simulink model "benchmark_16bus_base_scenario"  (R2021a)
settings: Solver=ode4  StartTime=0.0  StopTime=5  FixedStep=Ts  MaxStep=50e-6  RelTol=1e-3
values from neighbouring files (symbols this model uses):
  Ctrl_Delay = 100e-6    (= 0.0001)    [init_anon.m]
  Pnom1 = 1330e6    (= 1330000000)    [init_anon.m]
  Pnom3 = 1e9    (= 1000000000)    [init_anon.m]
  Pnom4 = 64.4e6    (= 64400000)    [init_anon.m]
  Pnom5 = 19e6    (= 19000000)    [init_anon.m]
  Pnom6 = 450e6    (= 450000000)    [init_anon.m]
  Snom1 = 1e6*sqrt(1330^2 + (0.3*1330)^2)    [init_anon.m]
  Snom3 = 1044e6    (= 1044000000)    [init_anon.m]
  Snom4 = 1e6*sqrt(64.4^2 + (0.3*64.4)^2)    [init_anon.m]
  Snom5 = 1e6*sqrt(19^2 + (0.3*19)^2)    [init_anon.m]
  Snom6 = 1e6*sqrt(450^2 + (0.3*450)^2)    [init_anon.m]
  Ts = 5e-6    (= 5e-06)    [init_anon.m]
  wb = 2*pi*50    (= 314.159265359)    [init_anon.m]
  wcc = 1200    [init_anon.m]
  wlpf = 300    [init_anon.m]
  wp = 10    [init_anon.m]
  wv = 50    [init_anon.m]
  Zb = Ub^2/Sb    [init_anon.m]
undefined symbols (not defined in the file or in its folder): fb, Ib2, Ki_CC, Ki_i, Kp_CC, Kp_i, Kp_Rvi_pu, Lc_eq, Lf_pu, Rc_eq, Sb, Va0, Vb0, Vb1, Vb2, Vc0, Vm0, Vm0_d, Vm0_q, VSC01_id0, Vvsc0
libraries: spsGroundLib x135, spsParallelRLCBranchLib x132, Control_Lib x120, spsSeriesRLCBranchLib x66, spsThreePhaseSourceLib x22, spsThreePhaseBreakerLib x20, eeGeneralControl x20, slpidlib x15, spsLoadFlowBusLib x13, spsThreePhaseVIMeasurementLib x12, spsThreePhaseTransformerTwoWindingsLib x11, spsUniversalBridgeLib x10
(part 3 of 9)

== system benchmark_16bus_base_scenario/Subsystem15 ==
  Ground{,1..5} (6 alike) : spsGroundLib/Ground  LConnTagsString=a
  Parallel RLC Branch{,1..5} (6 alike) : spsParallelRLCBranchLib/Parallel RLC Branch  LConnTagsString=a  RConnTagsString=__new0  BranchType=C  Resistance=1  Inductance=1e-3  SetiL0=off  InitialCurrent=0  Capacitance=C  Setx0=off  InitialVoltage=0  Measurements=None
  Series RLC Branch : spsSeriesRLCBranchLib/Series RLC Branch  LConnTagsString=__new0  RConnTagsString=__new0  BranchType=RL  Resistance=R  Inductance=L  SetiL0=off  InitialCurrent=0  Capacitance=1e-6  Setx0=off  InitialVoltage=0  Measurements=None
  Series RLC Branch3 : spsSeriesRLCBranchLib/Series RLC Branch  LConnTagsString=__new0  RConnTagsString=__new0  BranchType=RL  Resistance=R  Inductance=L  SetiL0=off  InitialCurrent=0  Capacitance=1e-6  Setx0=off  InitialVoltage=0  Measurements=None
  Series RLC Branch6 : spsSeriesRLCBranchLib/Series RLC Branch  LConnTagsString=__new0  RConnTagsString=__new0  BranchType=RL  Resistance=R  Inductance=L  SetiL0=off  InitialCurrent=0  Capacitance=1e-6  Setx0=off  InitialVoltage=0  Measurements=None
  A : PMIOPort  Side=Left
  a : PMIOPort  Port=2  Side=Right
  B : PMIOPort  Port=3  Side=Left
  b : PMIOPort  Port=4  Side=Right
  C : PMIOPort  Port=5  Side=Left
  c : PMIOPort  Port=6  Side=Right
  connections:
  Ground5/LConn1 -- Parallel RLC Branch5/RConn1
  Ground4/LConn1 -- Parallel RLC Branch4/RConn1
  Series RLC Branch6/RConn1 -- Parallel RLC Branch5/LConn1 -- c/RConn1
  Series RLC Branch6/LConn1 -- Parallel RLC Branch4/LConn1 -- C/RConn1
  Ground3/LConn1 -- Parallel RLC Branch3/RConn1
  Ground2/LConn1 -- Parallel RLC Branch2/RConn1
  Series RLC Branch3/RConn1 -- Parallel RLC Branch3/LConn1 -- b/RConn1
  Series RLC Branch3/LConn1 -- Parallel RLC Branch2/LConn1 -- B/RConn1
  Parallel RLC Branch1/LConn1 -- a/RConn1 -- Series RLC Branch/RConn1
  Ground/LConn1 -- Parallel RLC Branch/RConn1
  Parallel RLC Branch/LConn1 -- A/RConn1 -- Series RLC Branch/LConn1
  Ground1/LConn1 -- Parallel RLC Branch1/RConn1

== system benchmark_16bus_base_scenario/Subsystem16 ==
  Ground{,1..5} (6 alike) : spsGroundLib/Ground  LConnTagsString=a
  Parallel RLC Branch{,1..5} (6 alike) : spsParallelRLCBranchLib/Parallel RLC Branch  LConnTagsString=a  RConnTagsString=__new0  BranchType=C  Resistance=1  Inductance=1e-3  SetiL0=off  InitialCurrent=0  Capacitance=C  Setx0=off  InitialVoltage=0  Measurements=None
  Series RLC Branch : spsSeriesRLCBranchLib/Series RLC Branch  LConnTagsString=__new0  RConnTagsString=__new0  BranchType=RL  Resistance=R  Inductance=L  SetiL0=off  InitialCurrent=0  Capacitance=1e-6  Setx0=off  InitialVoltage=0  Measurements=None
  Series RLC Branch3 : spsSeriesRLCBranchLib/Series RLC Branch  LConnTagsString=__new0  RConnTagsString=__new0  BranchType=RL  Resistance=R  Inductance=L  SetiL0=off  InitialCurrent=0  Capacitance=1e-6  Setx0=off  InitialVoltage=0  Measurements=None
  Series RLC Branch6 : spsSeriesRLCBranchLib/Series RLC Branch  LConnTagsString=__new0  RConnTagsString=__new0  BranchType=RL  Resistance=R  Inductance=L  SetiL0=off  InitialCurrent=0  Capacitance=1e-6  Setx0=off  InitialVoltage=0  Measurements=None
  A : PMIOPort  Side=Left
  a : PMIOPort  Port=2  Side=Right
  B : PMIOPort  Port=3  Side=Left
  b : PMIOPort  Port=4  Side=Right
  C : PMIOPort  Port=5  Side=Left
  c : PMIOPort  Port=6  Side=Right
  connections:
  Ground1/LConn1 -- Parallel RLC Branch1/RConn1
  Series RLC Branch/LConn1 -- A/RConn1 -- Parallel RLC Branch/LConn1
  Ground/LConn1 -- Parallel RLC Branch/RConn1
  Series RLC Branch/RConn1 -- a/RConn1 -- Parallel RLC Branch1/LConn1
  B/RConn1 -- Parallel RLC Branch2/LConn1 -- Series RLC Branch3/LConn1
  b/RConn1 -- Parallel RLC Branch3/LConn1 -- Series RLC Branch3/RConn1
  Ground2/LConn1 -- Parallel RLC Branch2/RConn1
  Ground3/LConn1 -- Parallel RLC Branch3/RConn1
  C/RConn1 -- Parallel RLC Branch4/LConn1 -- Series RLC Branch6/LConn1
  c/RConn1 -- Parallel RLC Branch5/LConn1 -- Series RLC Branch6/RConn1
  Ground4/LConn1 -- Parallel RLC Branch4/RConn1
  Ground5/LConn1 -- Parallel RLC Branch5/RConn1

== system benchmark_16bus_base_scenario/Subsystem17 ==
  Ground{,1..5} (6 alike) : spsGroundLib/Ground  LConnTagsString=a
  Parallel RLC Branch{,1..5} (6 alike) : spsParallelRLCBranchLib/Parallel RLC Branch  LConnTagsString=a  RConnTagsString=__new0  BranchType=C  Resistance=1  Inductance=1e-3  SetiL0=off  InitialCurrent=0  Capacitance=C  Setx0=off  InitialVoltage=0  Measurements=None
  Series RLC Branch : spsSeriesRLCBranchLib/Series RLC Branch  LConnTagsString=__new0  RConnTagsString=__new0  BranchType=RL  Resistance=R  Inductance=L  SetiL0=off  InitialCurrent=0  Capacitance=1e-6  Setx0=off  InitialVoltage=0  Measurements=None
  Series RLC Branch3 : spsSeriesRLCBranchLib/Series RLC Branch  LConnTagsString=__new0  RConnTagsString=__new0  BranchType=RL  Resistance=R  Inductance=L  SetiL0=off  InitialCurrent=0  Capacitance=1e-6  Setx0=off  InitialVoltage=0  Measurements=None
  Series RLC Branch6 : spsSeriesRLCBranchLib/Series RLC Branch  LConnTagsString=__new0  RConnTagsString=__new0  BranchType=RL  Resistance=R  Inductance=L  SetiL0=off  InitialCurrent=0  Capacitance=1e-6  Setx0=off  InitialVoltage=0  Measurements=None
  A : PMIOPort  Side=Left
  a : PMIOPort  Port=2  Side=Right
  B : PMIOPort  Port=3  Side=Left
  b : PMIOPort  Port=4  Side=Right
  C : PMIOPort  Port=5  Side=Left
  c : PMIOPort  Port=6  Side=Right
  connections:
  Ground5/LConn1 -- Parallel RLC Branch5/RConn1
  Ground4/LConn1 -- Parallel RLC Branch4/RConn1
  Series RLC Branch6/RConn1 -- Parallel RLC Branch5/LConn1 -- c/RConn1
  Series RLC Branch6/LConn1 -- Parallel RLC Branch4/LConn1 -- C/RConn1
  Ground3/LConn1 -- Parallel RLC Branch3/RConn1
  Ground2/LConn1 -- Parallel RLC Branch2/RConn1
  Series RLC Branch3/RConn1 -- Parallel RLC Branch3/LConn1 -- b/RConn1
  Series RLC Branch3/LConn1 -- Parallel RLC Branch2/LConn1 -- B/RConn1
  Parallel RLC Branch1/LConn1 -- a/RConn1 -- Series RLC Branch/RConn1
  Ground/LConn1 -- Parallel RLC Branch/RConn1
  Parallel RLC Branch/LConn1 -- A/RConn1 -- Series RLC Branch/LConn1
  Ground1/LConn1 -- Parallel RLC Branch1/RConn1

== system benchmark_16bus_base_scenario/Subsystem18 ==
  Ground{,1..5} (6 alike) : spsGroundLib/Ground  LConnTagsString=a
  Parallel RLC Branch{,1..5} (6 alike) : spsParallelRLCBranchLib/Parallel RLC Branch  LConnTagsString=a  RConnTagsString=__new0  BranchType=C  Resistance=1  Inductance=1e-3  SetiL0=off  InitialCurrent=0  Capacitance=C  Setx0=off  InitialVoltage=0  Measurements=None
  Series RLC Branch : spsSeriesRLCBranchLib/Series RLC Branch  LConnTagsString=__new0  RConnTagsString=__new0  BranchType=RL  Resistance=R  Inductance=L  SetiL0=off  InitialCurrent=0  Capacitance=1e-6  Setx0=off  InitialVoltage=0  Measurements=None
  Series RLC Branch3 : spsSeriesRLCBranchLib/Series RLC Branch  LConnTagsString=__new0  RConnTagsString=__new0  BranchType=RL  Resistance=R  Inductance=L  SetiL0=off  InitialCurrent=0  Capacitance=1e-6  Setx0=off  InitialVoltage=0  Measurements=None
  Series RLC Branch6 : spsSeriesRLCBranchLib/Series RLC Branch  LConnTagsString=__new0  RConnTagsString=__new0  BranchType=RL  Resistance=R  Inductance=L  SetiL0=off  InitialCurrent=0  Capacitance=1e-6  Setx0=off  InitialVoltage=0  Measurements=None
  A : PMIOPort  Side=Left
  a : PMIOPort  Port=2  Side=Right
  B : PMIOPort  Port=3  Side=Left
  b : PMIOPort  Port=4  Side=Right
  C : PMIOPort  Port=5  Side=Left
  c : PMIOPort  Port=6  Side=Right
  connections:
  Ground5/LConn1 -- Parallel RLC Branch5/RConn1
  Ground4/LConn1 -- Parallel RLC Branch4/RConn1
  Series RLC Branch6/RConn1 -- Parallel RLC Branch5/LConn1 -- c/RConn1
  Series RLC Branch6/LConn1 -- Parallel RLC Branch4/LConn1 -- C/RConn1
  Ground3/LConn1 -- Parallel RLC Branch3/RConn1
  Ground2/LConn1 -- Parallel RLC Branch2/RConn1
  Series RLC Branch3/RConn1 -- Parallel RLC Branch3/LConn1 -- b/RConn1
  Series RLC Branch3/LConn1 -- Parallel RLC Branch2/LConn1 -- B/RConn1
  Parallel RLC Branch1/LConn1 -- a/RConn1 -- Series RLC Branch/RConn1
  Ground/LConn1 -- Parallel RLC Branch/RConn1
  Parallel RLC Branch/LConn1 -- A/RConn1 -- Series RLC Branch/LConn1
  Ground1/LConn1 -- Parallel RLC Branch1/RConn1

== system benchmark_16bus_base_scenario/Subsystem19 ==
  Ground{,1..5} (6 alike) : spsGroundLib/Ground  LConnTagsString=a
  Parallel RLC Branch{,1..5} (6 alike) : spsParallelRLCBranchLib/Parallel RLC Branch  LConnTagsString=a  RConnTagsString=__new0  BranchType=C  Resistance=1  Inductance=1e-3  SetiL0=off  InitialCurrent=0  Capacitance=C  Setx0=off  InitialVoltage=0  Measurements=None
  Series RLC Branch : spsSeriesRLCBranchLib/Series RLC Branch  LConnTagsString=__new0  RConnTagsString=__new0  BranchType=RL  Resistance=R  Inductance=L  SetiL0=off  InitialCurrent=0  Capacitance=1e-6  Setx0=off  InitialVoltage=0  Measurements=None
  Series RLC Branch3 : spsSeriesRLCBranchLib/Series RLC Branch  LConnTagsString=__new0  RConnTagsString=__new0  BranchType=RL  Resistance=R  Inductance=L  SetiL0=off  InitialCurrent=0  Capacitance=1e-6  Setx0=off  InitialVoltage=0  Measurements=None
  Series RLC Branch6 : spsSeriesRLCBranchLib/Series RLC Branch  LConnTagsString=__new0  RConnTagsString=__new0  BranchType=RL  Resistance=R  Inductance=L  SetiL0=off  InitialCurrent=0  Capacitance=1e-6  Setx0=off  InitialVoltage=0  Measurements=None
  A : PMIOPort  Side=Left
  a : PMIOPort  Port=2  Side=Right
  B : PMIOPort  Port=3  Side=Left
  b : PMIOPort  Port=4  Side=Right
  C : PMIOPort  Port=5  Side=Left
  c : PMIOPort  Port=6  Side=Right
  connections:
  Ground1/LConn1 -- Parallel RLC Branch1/RConn1
  Series RLC Branch/LConn1 -- A/RConn1 -- Parallel RLC Branch/LConn1
  Ground/LConn1 -- Parallel RLC Branch/RConn1
  Series RLC Branch/RConn1 -- a/RConn1 -- Parallel RLC Branch1/LConn1
  B/RConn1 -- Parallel RLC Branch2/LConn1 -- Series RLC Branch3/LConn1
  b/RConn1 -- Parallel RLC Branch3/LConn1 -- Series RLC Branch3/RConn1
  Ground2/LConn1 -- Parallel RLC Branch2/RConn1
  Ground3/LConn1 -- Parallel RLC Branch3/RConn1
  C/RConn1 -- Parallel RLC Branch4/LConn1 -- Series RLC Branch6/LConn1
  c/RConn1 -- Parallel RLC Branch5/LConn1 -- Series RLC Branch6/RConn1
  Ground4/LConn1 -- Parallel RLC Branch4/RConn1
  Ground5/LConn1 -- Parallel RLC Branch5/RConn1

== system benchmark_16bus_base_scenario/Subsystem20 ==
  Ground{,1..5} (6 alike) : spsGroundLib/Ground  LConnTagsString=a
  Parallel RLC Branch{,1..5} (6 alike) : spsParallelRLCBranchLib/Parallel RLC Branch  LConnTagsString=a  RConnTagsString=__new0  BranchType=C  Resistance=1  Inductance=1e-3  SetiL0=off  InitialCurrent=0  Capacitance=C  Setx0=off  InitialVoltage=0  Measurements=None
  Series RLC Branch : spsSeriesRLCBranchLib/Series RLC Branch  LConnTagsString=__new0  RConnTagsString=__new0  BranchType=RL  Resistance=R  Inductance=L  SetiL0=off  InitialCurrent=0  Capacitance=1e-6  Setx0=off  InitialVoltage=0  Measurements=None
  Series RLC Branch3 : spsSeriesRLCBranchLib/Series RLC Branch  LConnTagsString=__new0  RConnTagsString=__new0  BranchType=RL  Resistance=R  Inductance=L  SetiL0=off  InitialCurrent=0  Capacitance=1e-6  Setx0=off  InitialVoltage=0  Measurements=None
  Series RLC Branch6 : spsSeriesRLCBranchLib/Series RLC Branch  LConnTagsString=__new0  RConnTagsString=__new0  BranchType=RL  Resistance=R  Inductance=L  SetiL0=off  InitialCurrent=0  Capacitance=1e-6  Setx0=off  InitialVoltage=0  Measurements=None
  A : PMIOPort  Side=Left
  a : PMIOPort  Port=2  Side=Right
  B : PMIOPort  Port=3  Side=Left
  b : PMIOPort  Port=4  Side=Right
  C : PMIOPort  Port=5  Side=Left
  c : PMIOPort  Port=6  Side=Right
  connections:
  Ground1/LConn1 -- Parallel RLC Branch1/RConn1
  Series RLC Branch/LConn1 -- A/RConn1 -- Parallel RLC Branch/LConn1
  Ground/LConn1 -- Parallel RLC Branch/RConn1
  Series RLC Branch/RConn1 -- a/RConn1 -- Parallel RLC Branch1/LConn1
  B/RConn1 -- Parallel RLC Branch2/LConn1 -- Series RLC Branch3/LConn1
  b/RConn1 -- Parallel RLC Branch3/LConn1 -- Series RLC Branch3/RConn1
  Ground2/LConn1 -- Parallel RLC Branch2/RConn1
  Ground3/LConn1 -- Parallel RLC Branch3/RConn1
  C/RConn1 -- Parallel RLC Branch4/LConn1 -- Series RLC Branch6/LConn1
  c/RConn1 -- Parallel RLC Branch5/LConn1 -- Series RLC Branch6/RConn1
  Ground4/LConn1 -- Parallel RLC Branch4/RConn1
  Ground5/LConn1 -- Parallel RLC Branch5/RConn1

== system benchmark_16bus_base_scenario/Subsystem21 ==
  Ground{,1..5} (6 alike) : spsGroundLib/Ground  LConnTagsString=a
  Parallel RLC Branch{,1..5} (6 alike) : spsParallelRLCBranchLib/Parallel RLC Branch  LConnTagsString=a  RConnTagsString=__new0  BranchType=C  Resistance=1  Inductance=1e-3  SetiL0=off  InitialCurrent=0  Capacitance=C  Setx0=off  InitialVoltage=0  Measurements=None
  Series RLC Branch : spsSeriesRLCBranchLib/Series RLC Branch  LConnTagsString=__new0  RConnTagsString=__new0  BranchType=RL  Resistance=R  Inductance=L  SetiL0=off  InitialCurrent=0  Capacitance=1e-6  Setx0=off  InitialVoltage=0  Measurements=None
  Series RLC Branch3 : spsSeriesRLCBranchLib/Series RLC Branch  LConnTagsString=__new0  RConnTagsString=__new0  BranchType=RL  Resistance=R  Inductance=L  SetiL0=off  InitialCurrent=0  Capacitance=1e-6  Setx0=off  InitialVoltage=0  Measurements=None
  Series RLC Branch6 : spsSeriesRLCBranchLib/Series RLC Branch  LConnTagsString=__new0  RConnTagsString=__new0  BranchType=RL  Resistance=R  Inductance=L  SetiL0=off  InitialCurrent=0  Capacitance=1e-6  Setx0=off  InitialVoltage=0  Measurements=None
  A : PMIOPort  Side=Left
  a : PMIOPort  Port=2  Side=Right
  B : PMIOPort  Port=3  Side=Left
  b : PMIOPort  Port=4  Side=Right
  C : PMIOPort  Port=5  Side=Left
  c : PMIOPort  Port=6  Side=Right
  connections:
  Ground5/LConn1 -- Parallel RLC Branch5/RConn1
  Ground4/LConn1 -- Parallel RLC Branch4/RConn1
  Series RLC Branch6/RConn1 -- Parallel RLC Branch5/LConn1 -- c/RConn1
  Series RLC Branch6/LConn1 -- Parallel RLC Branch4/LConn1 -- C/RConn1
  Ground3/LConn1 -- Parallel RLC Branch3/RConn1
  Ground2/LConn1 -- Parallel RLC Branch2/RConn1
  Series RLC Branch3/RConn1 -- Parallel RLC Branch3/LConn1 -- b/RConn1
  Series RLC Branch3/LConn1 -- Parallel RLC Branch2/LConn1 -- B/RConn1
  Parallel RLC Branch1/LConn1 -- a/RConn1 -- Series RLC Branch/RConn1
  Ground/LConn1 -- Parallel RLC Branch/RConn1
  Parallel RLC Branch/LConn1 -- A/RConn1 -- Series RLC Branch/LConn1
  Ground1/LConn1 -- Parallel RLC Branch1/RConn1

== system benchmark_16bus_base_scenario/Subsystem22 ==
  Ground{,1..5} (6 alike) : spsGroundLib/Ground  LConnTagsString=a
  Parallel RLC Branch{,1..5} (6 alike) : spsParallelRLCBranchLib/Parallel RLC Branch  LConnTagsString=a  RConnTagsString=__new0  BranchType=C  Resistance=1  Inductance=1e-3  SetiL0=off  InitialCurrent=0  Capacitance=C  Setx0=off  InitialVoltage=0  Measurements=None
  Series RLC Branch : spsSeriesRLCBranchLib/Series RLC Branch  LConnTagsString=__new0  RConnTagsString=__new0  BranchType=RL  Resistance=R  Inductance=L  SetiL0=off  InitialCurrent=0  Capacitance=1e-6  Setx0=off  InitialVoltage=0  Measurements=None
  Series RLC Branch3 : spsSeriesRLCBranchLib/Series RLC Branch  LConnTagsString=__new0  RConnTagsString=__new0  BranchType=RL  Resistance=R  Inductance=L  SetiL0=off  InitialCurrent=0  Capacitance=1e-6  Setx0=off  InitialVoltage=0  Measurements=None
  Series RLC Branch6 : spsSeriesRLCBranchLib/Series RLC Branch  LConnTagsString=__new0  RConnTagsString=__new0  BranchType=RL  Resistance=R  Inductance=L  SetiL0=off  InitialCurrent=0  Capacitance=1e-6  Setx0=off  InitialVoltage=0  Measurements=None
  A : PMIOPort  Side=Left
  a : PMIOPort  Port=2  Side=Right
  B : PMIOPort  Port=3  Side=Left
  b : PMIOPort  Port=4  Side=Right
  C : PMIOPort  Port=5  Side=Left
  c : PMIOPort  Port=6  Side=Right
  connections:
  Ground5/LConn1 -- Parallel RLC Branch5/RConn1
  Ground4/LConn1 -- Parallel RLC Branch4/RConn1
  Series RLC Branch6/RConn1 -- Parallel RLC Branch5/LConn1 -- c/RConn1
  Series RLC Branch6/LConn1 -- Parallel RLC Branch4/LConn1 -- C/RConn1
  Ground3/LConn1 -- Parallel RLC Branch3/RConn1
  Ground2/LConn1 -- Parallel RLC Branch2/RConn1
  Series RLC Branch3/RConn1 -- Parallel RLC Branch3/LConn1 -- b/RConn1
  Series RLC Branch3/LConn1 -- Parallel RLC Branch2/LConn1 -- B/RConn1
  Parallel RLC Branch1/LConn1 -- a/RConn1 -- Series RLC Branch/RConn1
  Ground/LConn1 -- Parallel RLC Branch/RConn1
  Parallel RLC Branch/LConn1 -- A/RConn1 -- Series RLC Branch/LConn1
  Ground1/LConn1 -- Parallel RLC Branch1/RConn1

== system benchmark_16bus_base_scenario/Subsystem23 ==
  Ground{,1..5} (6 alike) : spsGroundLib/Ground  LConnTagsString=a
  Parallel RLC Branch{,1..5} (6 alike) : spsParallelRLCBranchLib/Parallel RLC Branch  LConnTagsString=a  RConnTagsString=__new0  BranchType=C  Resistance=1  Inductance=1e-3  SetiL0=off  InitialCurrent=0  Capacitance=C  Setx0=off  InitialVoltage=0  Measurements=None
  Series RLC Branch : spsSeriesRLCBranchLib/Series RLC Branch  LConnTagsString=__new0  RConnTagsString=__new0  BranchType=RL  Resistance=R  Inductance=L  SetiL0=off  InitialCurrent=0  Capacitance=1e-6  Setx0=off  InitialVoltage=0  Measurements=None
  Series RLC Branch3 : spsSeriesRLCBranchLib/Series RLC Branch  LConnTagsString=__new0  RConnTagsString=__new0  BranchType=RL  Resistance=R  Inductance=L  SetiL0=off  InitialCurrent=0  Capacitance=1e-6  Setx0=off  InitialVoltage=0  Measurements=None
  Series RLC Branch6 : spsSeriesRLCBranchLib/Series RLC Branch  LConnTagsString=__new0  RConnTagsString=__new0  BranchType=RL  Resistance=R  Inductance=L  SetiL0=off  InitialCurrent=0  Capacitance=1e-6  Setx0=off  InitialVoltage=0  Measurements=None
  A : PMIOPort  Side=Left
  a : PMIOPort  Port=2  Side=Right
  B : PMIOPort  Port=3  Side=Left
  b : PMIOPort  Port=4  Side=Right
  C : PMIOPort  Port=5  Side=Left
  c : PMIOPort  Port=6  Side=Right
  connections:
  Ground1/LConn1 -- Parallel RLC Branch1/RConn1
  Series RLC Branch/LConn1 -- A/RConn1 -- Parallel RLC Branch/LConn1
  Ground/LConn1 -- Parallel RLC Branch/RConn1
  Series RLC Branch/RConn1 -- a/RConn1 -- Parallel RLC Branch1/LConn1
  B/RConn1 -- Parallel RLC Branch2/LConn1 -- Series RLC Branch3/LConn1
  b/RConn1 -- Parallel RLC Branch3/LConn1 -- Series RLC Branch3/RConn1
  Ground2/LConn1 -- Parallel RLC Branch2/RConn1
  Ground3/LConn1 -- Parallel RLC Branch3/RConn1
  C/RConn1 -- Parallel RLC Branch4/LConn1 -- Series RLC Branch6/LConn1
  c/RConn1 -- Parallel RLC Branch5/LConn1 -- Series RLC Branch6/RConn1
  Ground4/LConn1 -- Parallel RLC Branch4/RConn1
  Ground5/LConn1 -- Parallel RLC Branch5/RConn1

== system benchmark_16bus_base_scenario/Subsystem24 ==
  Ground{,1..5} (6 alike) : spsGroundLib/Ground  LConnTagsString=a
  Parallel RLC Branch{,1..5} (6 alike) : spsParallelRLCBranchLib/Parallel RLC Branch  LConnTagsString=a  RConnTagsString=__new0  BranchType=C  Resistance=1  Inductance=1e-3  SetiL0=off  InitialCurrent=0  Capacitance=C  Setx0=off  InitialVoltage=0  Measurements=None
  Series RLC Branch : spsSeriesRLCBranchLib/Series RLC Branch  LConnTagsString=__new0  RConnTagsString=__new0  BranchType=RL  Resistance=R  Inductance=L  SetiL0=off  InitialCurrent=0  Capacitance=1e-6  Setx0=off  InitialVoltage=0  Measurements=None
  Series RLC Branch3 : spsSeriesRLCBranchLib/Series RLC Branch  LConnTagsString=__new0  RConnTagsString=__new0  BranchType=RL  Resistance=R  Inductance=L  SetiL0=off  InitialCurrent=0  Capacitance=1e-6  Setx0=off  InitialVoltage=0  Measurements=None
  Series RLC Branch6 : spsSeriesRLCBranchLib/Series RLC Branch  LConnTagsString=__new0  RConnTagsString=__new0  BranchType=RL  Resistance=R  Inductance=L  SetiL0=off  InitialCurrent=0  Capacitance=1e-6  Setx0=off  InitialVoltage=0  Measurements=None
  A : PMIOPort  Side=Left
  a : PMIOPort  Port=2  Side=Right
  B : PMIOPort  Port=3  Side=Left
  b : PMIOPort  Port=4  Side=Right
  C : PMIOPort  Port=5  Side=Left
  c : PMIOPort  Port=6  Side=Right
  connections:
  Ground5/LConn1 -- Parallel RLC Branch5/RConn1
  Ground4/LConn1 -- Parallel RLC Branch4/RConn1
  Series RLC Branch6/RConn1 -- Parallel RLC Branch5/LConn1 -- c/RConn1
  Series RLC Branch6/LConn1 -- Parallel RLC Branch4/LConn1 -- C/RConn1
  Ground3/LConn1 -- Parallel RLC Branch3/RConn1
  Ground2/LConn1 -- Parallel RLC Branch2/RConn1
  Series RLC Branch3/RConn1 -- Parallel RLC Branch3/LConn1 -- b/RConn1
  Series RLC Branch3/LConn1 -- Parallel RLC Branch2/LConn1 -- B/RConn1
  Parallel RLC Branch1/LConn1 -- a/RConn1 -- Series RLC Branch/RConn1
  Ground/LConn1 -- Parallel RLC Branch/RConn1
  Parallel RLC Branch/LConn1 -- A/RConn1 -- Series RLC Branch/LConn1
  Ground1/LConn1 -- Parallel RLC Branch1/RConn1

== system benchmark_16bus_base_scenario/Subsystem25 ==
  Ground{,1..5} (6 alike) : spsGroundLib/Ground  LConnTagsString=a
  Parallel RLC Branch{,1..5} (6 alike) : spsParallelRLCBranchLib/Parallel RLC Branch  LConnTagsString=a  RConnTagsString=__new0  BranchType=C  Resistance=1  Inductance=1e-3  SetiL0=off  InitialCurrent=0  Capacitance=C  Setx0=off  InitialVoltage=0  Measurements=None
  Series RLC Branch : spsSeriesRLCBranchLib/Series RLC Branch  LConnTagsString=__new0  RConnTagsString=__new0  BranchType=RL  Resistance=R  Inductance=L  SetiL0=off  InitialCurrent=0  Capacitance=1e-6  Setx0=off  InitialVoltage=0  Measurements=None
  Series RLC Branch3 : spsSeriesRLCBranchLib/Series RLC Branch  LConnTagsString=__new0  RConnTagsString=__new0  BranchType=RL  Resistance=R  Inductance=L  SetiL0=off  InitialCurrent=0  Capacitance=1e-6  Setx0=off  InitialVoltage=0  Measurements=None
  Series RLC Branch6 : spsSeriesRLCBranchLib/Series RLC Branch  LConnTagsString=__new0  RConnTagsString=__new0  BranchType=RL  Resistance=R  Inductance=L  SetiL0=off  InitialCurrent=0  Capacitance=1e-6  Setx0=off  InitialVoltage=0  Measurements=None
  A : PMIOPort  Side=Left
  a : PMIOPort  Port=2  Side=Right
  B : PMIOPort  Port=3  Side=Left
  b : PMIOPort  Port=4  Side=Right
  C : PMIOPort  Port=5  Side=Left
  c : PMIOPort  Port=6  Side=Right
  connections:
  Ground1/LConn1 -- Parallel RLC Branch1/RConn1
  Series RLC Branch/LConn1 -- A/RConn1 -- Parallel RLC Branch/LConn1
  Ground/LConn1 -- Parallel RLC Branch/RConn1
  Series RLC Branch/RConn1 -- a/RConn1 -- Parallel RLC Branch1/LConn1
  B/RConn1 -- Parallel RLC Branch2/LConn1 -- Series RLC Branch3/LConn1
  b/RConn1 -- Parallel RLC Branch3/LConn1 -- Series RLC Branch3/RConn1
  Ground2/LConn1 -- Parallel RLC Branch2/RConn1
  Ground3/LConn1 -- Parallel RLC Branch3/RConn1
  C/RConn1 -- Parallel RLC Branch4/LConn1 -- Series RLC Branch6/LConn1
  c/RConn1 -- Parallel RLC Branch5/LConn1 -- Series RLC Branch6/RConn1
  Ground4/LConn1 -- Parallel RLC Branch4/RConn1
  Ground5/LConn1 -- Parallel RLC Branch5/RConn1

== system benchmark_16bus_base_scenario/Subsystem26 ==
  Ground{,1..5} (6 alike) : spsGroundLib/Ground  LConnTagsString=a
  Parallel RLC Branch{,1..5} (6 alike) : spsParallelRLCBranchLib/Parallel RLC Branch  LConnTagsString=a  RConnTagsString=__new0  BranchType=C  Resistance=1  Inductance=1e-3  SetiL0=off  InitialCurrent=0  Capacitance=C  Setx0=off  InitialVoltage=0  Measurements=None
  Series RLC Branch : spsSeriesRLCBranchLib/Series RLC Branch  LConnTagsString=__new0  RConnTagsString=__new0  BranchType=RL  Resistance=R  Inductance=L  SetiL0=off  InitialCurrent=0  Capacitance=1e-6  Setx0=off  InitialVoltage=0  Measurements=None
  Series RLC Branch3 : spsSeriesRLCBranchLib/Series RLC Branch  LConnTagsString=__new0  RConnTagsString=__new0  BranchType=RL  Resistance=R  Inductance=L  SetiL0=off  InitialCurrent=0  Capacitance=1e-6  Setx0=off  InitialVoltage=0  Measurements=None
  Series RLC Branch6 : spsSeriesRLCBranchLib/Series RLC Branch  LConnTagsString=__new0  RConnTagsString=__new0  BranchType=RL  Resistance=R  Inductance=L  SetiL0=off  InitialCurrent=0  Capacitance=1e-6  Setx0=off  InitialVoltage=0  Measurements=None
  A : PMIOPort  Side=Left
  a : PMIOPort  Port=2  Side=Right
  B : PMIOPort  Port=3  Side=Left
  b : PMIOPort  Port=4  Side=Right
  C : PMIOPort  Port=5  Side=Left
  c : PMIOPort  Port=6  Side=Right
  connections:
  Ground5/LConn1 -- Parallel RLC Branch5/RConn1
  Ground4/LConn1 -- Parallel RLC Branch4/RConn1
  Series RLC Branch6/RConn1 -- Parallel RLC Branch5/LConn1 -- c/RConn1
  Series RLC Branch6/LConn1 -- Parallel RLC Branch4/LConn1 -- C/RConn1
  Ground3/LConn1 -- Parallel RLC Branch3/RConn1
  Ground2/LConn1 -- Parallel RLC Branch2/RConn1
  Series RLC Branch3/RConn1 -- Parallel RLC Branch3/LConn1 -- b/RConn1
  Series RLC Branch3/LConn1 -- Parallel RLC Branch2/LConn1 -- B/RConn1
  Parallel RLC Branch1/LConn1 -- a/RConn1 -- Series RLC Branch/RConn1
  Ground/LConn1 -- Parallel RLC Branch/RConn1
  Parallel RLC Branch/LConn1 -- A/RConn1 -- Series RLC Branch/LConn1
  Ground1/LConn1 -- Parallel RLC Branch1/RConn1

== system benchmark_16bus_base_scenario/Subsystem27 ==
  Ground{,1..5} (6 alike) : spsGroundLib/Ground  LConnTagsString=a
  Parallel RLC Branch{,1..5} (6 alike) : spsParallelRLCBranchLib/Parallel RLC Branch  LConnTagsString=a  RConnTagsString=__new0  BranchType=C  Resistance=1  Inductance=1e-3  SetiL0=off  InitialCurrent=0  Capacitance=C  Setx0=off  InitialVoltage=0  Measurements=None
  Series RLC Branch : spsSeriesRLCBranchLib/Series RLC Branch  LConnTagsString=__new0  RConnTagsString=__new0  BranchType=RL  Resistance=R  Inductance=L  SetiL0=off  InitialCurrent=0  Capacitance=1e-6  Setx0=off  InitialVoltage=0  Measurements=None
  Series RLC Branch3 : spsSeriesRLCBranchLib/Series RLC Branch  LConnTagsString=__new0  RConnTagsString=__new0  BranchType=RL  Resistance=R  Inductance=L  SetiL0=off  InitialCurrent=0  Capacitance=1e-6  Setx0=off  InitialVoltage=0  Measurements=None
  Series RLC Branch6 : spsSeriesRLCBranchLib/Series RLC Branch  LConnTagsString=__new0  RConnTagsString=__new0  BranchType=RL  Resistance=R  Inductance=L  SetiL0=off  InitialCurrent=0  Capacitance=1e-6  Setx0=off  InitialVoltage=0  Measurements=None
  A : PMIOPort  Side=Left
  a : PMIOPort  Port=2  Side=Right
  B : PMIOPort  Port=3  Side=Left
  b : PMIOPort  Port=4  Side=Right
  C : PMIOPort  Port=5  Side=Left
  c : PMIOPort  Port=6  Side=Right
  connections:
  Ground1/LConn1 -- Parallel RLC Branch1/RConn1
  Series RLC Branch/LConn1 -- A/RConn1 -- Parallel RLC Branch/LConn1
  Ground/LConn1 -- Parallel RLC Branch/RConn1
  Series RLC Branch/RConn1 -- a/RConn1 -- Parallel RLC Branch1/LConn1
  B/RConn1 -- Parallel RLC Branch2/LConn1 -- Series RLC Branch3/LConn1
  b/RConn1 -- Parallel RLC Branch3/LConn1 -- Series RLC Branch3/RConn1
  Ground2/LConn1 -- Parallel RLC Branch2/RConn1
  Ground3/LConn1 -- Parallel RLC Branch3/RConn1
  C/RConn1 -- Parallel RLC Branch4/LConn1 -- Series RLC Branch6/LConn1
  c/RConn1 -- Parallel RLC Branch5/LConn1 -- Series RLC Branch6/RConn1
  Ground4/LConn1 -- Parallel RLC Branch4/RConn1
  Ground5/LConn1 -- Parallel RLC Branch5/RConn1

== system benchmark_16bus_base_scenario/Subsystem28 ==
  Ground{,1..5} (6 alike) : spsGroundLib/Ground  LConnTagsString=a
  Parallel RLC Branch{,1..5} (6 alike) : spsParallelRLCBranchLib/Parallel RLC Branch  LConnTagsString=a  RConnTagsString=__new0  BranchType=C  Resistance=1  Inductance=1e-3  SetiL0=off  InitialCurrent=0  Capacitance=C  Setx0=off  InitialVoltage=0  Measurements=None
  Series RLC Branch : spsSeriesRLCBranchLib/Series RLC Branch  LConnTagsString=__new0  RConnTagsString=__new0  BranchType=RL  Resistance=R  Inductance=L  SetiL0=off  InitialCurrent=0  Capacitance=1e-6  Setx0=off  InitialVoltage=0  Measurements=None
  Series RLC Branch3 : spsSeriesRLCBranchLib/Series RLC Branch  LConnTagsString=__new0  RConnTagsString=__new0  BranchType=RL  Resistance=R  Inductance=L  SetiL0=off  InitialCurrent=0  Capacitance=1e-6  Setx0=off  InitialVoltage=0  Measurements=None
  Series RLC Branch6 : spsSeriesRLCBranchLib/Series RLC Branch  LConnTagsString=__new0  RConnTagsString=__new0  BranchType=RL  Resistance=R  Inductance=L  SetiL0=off  InitialCurrent=0  Capacitance=1e-6  Setx0=off  InitialVoltage=0  Measurements=None
  A : PMIOPort  Side=Left
  a : PMIOPort  Port=2  Side=Right
  B : PMIOPort  Port=3  Side=Left
  b : PMIOPort  Port=4  Side=Right
  C : PMIOPort  Port=5  Side=Left
  c : PMIOPort  Port=6  Side=Right
  connections:
  Ground1/LConn1 -- Parallel RLC Branch1/RConn1
  Series RLC Branch/LConn1 -- A/RConn1 -- Parallel RLC Branch/LConn1
  Ground/LConn1 -- Parallel RLC Branch/RConn1
  Series RLC Branch/RConn1 -- a/RConn1 -- Parallel RLC Branch1/LConn1
  B/RConn1 -- Parallel RLC Branch2/LConn1 -- Series RLC Branch3/LConn1
  b/RConn1 -- Parallel RLC Branch3/LConn1 -- Series RLC Branch3/RConn1
  Ground2/LConn1 -- Parallel RLC Branch2/RConn1
  Ground3/LConn1 -- Parallel RLC Branch3/RConn1
  C/RConn1 -- Parallel RLC Branch4/LConn1 -- Series RLC Branch6/LConn1
  c/RConn1 -- Parallel RLC Branch5/LConn1 -- Series RLC Branch6/RConn1
  Ground4/LConn1 -- Parallel RLC Branch4/RConn1
  Ground5/LConn1 -- Parallel RLC Branch5/RConn1

== system benchmark_16bus_base_scenario/Subsystem29 ==
  Ground{,1..5} (6 alike) : spsGroundLib/Ground  LConnTagsString=a
  Parallel RLC Branch{,1..5} (6 alike) : spsParallelRLCBranchLib/Parallel RLC Branch  LConnTagsString=a  RConnTagsString=__new0  BranchType=C  Resistance=1  Inductance=1e-3  SetiL0=off  InitialCurrent=0  Capacitance=C  Setx0=off  InitialVoltage=0  Measurements=None
  Series RLC Branch : spsSeriesRLCBranchLib/Series RLC Branch  LConnTagsString=__new0  RConnTagsString=__new0  BranchType=RL  Resistance=R  Inductance=L  SetiL0=off  InitialCurrent=0  Capacitance=1e-6  Setx0=off  InitialVoltage=0  Measurements=None
  Series RLC Branch3 : spsSeriesRLCBranchLib/Series RLC Branch  LConnTagsString=__new0  RConnTagsString=__new0  BranchType=RL  Resistance=R  Inductance=L  SetiL0=off  InitialCurrent=0  Capacitance=1e-6  Setx0=off  InitialVoltage=0  Measurements=None
  Series RLC Branch6 : spsSeriesRLCBranchLib/Series RLC Branch  LConnTagsString=__new0  RConnTagsString=__new0  BranchType=RL  Resistance=R  Inductance=L  SetiL0=off  InitialCurrent=0  Capacitance=1e-6  Setx0=off  InitialVoltage=0  Measurements=None
  A : PMIOPort  Side=Left
  a : PMIOPort  Port=2  Side=Right
  B : PMIOPort  Port=3  Side=Left
  b : PMIOPort  Port=4  Side=Right
  C : PMIOPort  Port=5  Side=Left
  c : PMIOPort  Port=6  Side=Right
  connections:
  Ground5/LConn1 -- Parallel RLC Branch5/RConn1
  Ground4/LConn1 -- Parallel RLC Branch4/RConn1
  Series RLC Branch6/RConn1 -- Parallel RLC Branch5/LConn1 -- c/RConn1
  Series RLC Branch6/LConn1 -- Parallel RLC Branch4/LConn1 -- C/RConn1
  Ground3/LConn1 -- Parallel RLC Branch3/RConn1
  Ground2/LConn1 -- Parallel RLC Branch2/RConn1
  Series RLC Branch3/RConn1 -- Parallel RLC Branch3/LConn1 -- b/RConn1
  Series RLC Branch3/LConn1 -- Parallel RLC Branch2/LConn1 -- B/RConn1
  Parallel RLC Branch1/LConn1 -- a/RConn1 -- Series RLC Branch/RConn1
  Ground/LConn1 -- Parallel RLC Branch/RConn1
  Parallel RLC Branch/LConn1 -- A/RConn1 -- Series RLC Branch/LConn1
  Ground1/LConn1 -- Parallel RLC Branch1/RConn1

== system benchmark_16bus_base_scenario/Subsystem30 ==
  Ground{,1..5} (6 alike) : spsGroundLib/Ground  LConnTagsString=a
  Parallel RLC Branch{,1..5} (6 alike) : spsParallelRLCBranchLib/Parallel RLC Branch  LConnTagsString=a  RConnTagsString=__new0  BranchType=C  Resistance=1  Inductance=1e-3  SetiL0=off  InitialCurrent=0  Capacitance=C  Setx0=off  InitialVoltage=0  Measurements=None
  Series RLC Branch : spsSeriesRLCBranchLib/Series RLC Branch  LConnTagsString=__new0  RConnTagsString=__new0  BranchType=RL  Resistance=R  Inductance=L  SetiL0=off  InitialCurrent=0  Capacitance=1e-6  Setx0=off  InitialVoltage=0  Measurements=None
  Series RLC Branch3 : spsSeriesRLCBranchLib/Series RLC Branch  LConnTagsString=__new0  RConnTagsString=__new0  BranchType=RL  Resistance=R  Inductance=L  SetiL0=off  InitialCurrent=0  Capacitance=1e-6  Setx0=off  InitialVoltage=0  Measurements=None
  Series RLC Branch6 : spsSeriesRLCBranchLib/Series RLC Branch  LConnTagsString=__new0  RConnTagsString=__new0  BranchType=RL  Resistance=R  Inductance=L  SetiL0=off  InitialCurrent=0  Capacitance=1e-6  Setx0=off  InitialVoltage=0  Measurements=None
  A : PMIOPort  Side=Left
  a : PMIOPort  Port=2  Side=Right
  B : PMIOPort  Port=3  Side=Left
  b : PMIOPort  Port=4  Side=Right
  C : PMIOPort  Port=5  Side=Left
  c : PMIOPort  Port=6  Side=Right
  connections:
  Ground1/LConn1 -- Parallel RLC Branch1/RConn1
  Series RLC Branch/LConn1 -- A/RConn1 -- Parallel RLC Branch/LConn1
  Ground/LConn1 -- Parallel RLC Branch/RConn1
  Series RLC Branch/RConn1 -- a/RConn1 -- Parallel RLC Branch1/LConn1
  B/RConn1 -- Parallel RLC Branch2/LConn1 -- Series RLC Branch3/LConn1
  b/RConn1 -- Parallel RLC Branch3/LConn1 -- Series RLC Branch3/RConn1
  Ground2/LConn1 -- Parallel RLC Branch2/RConn1
  Ground3/LConn1 -- Parallel RLC Branch3/RConn1
  C/RConn1 -- Parallel RLC Branch4/LConn1 -- Series RLC Branch6/LConn1
  c/RConn1 -- Parallel RLC Branch5/LConn1 -- Series RLC Branch6/RConn1
  Ground4/LConn1 -- Parallel RLC Branch4/RConn1
  Ground5/LConn1 -- Parallel RLC Branch5/RConn1

== system benchmark_16bus_base_scenario/Subsystem9 ==
  Ground{,1..5} (6 alike) : spsGroundLib/Ground  LConnTagsString=a
  Parallel RLC Branch{,1..5} (6 alike) : spsParallelRLCBranchLib/Parallel RLC Branch  LConnTagsString=a  RConnTagsString=__new0  BranchType=C  Resistance=1  Inductance=1e-3  SetiL0=off  InitialCurrent=0  Capacitance=C  Setx0=off  InitialVoltage=0  Measurements=None
  Series RLC Branch : spsSeriesRLCBranchLib/Series RLC Branch  LConnTagsString=__new0  RConnTagsString=__new0  BranchType=RL  Resistance=R  Inductance=L  SetiL0=off  InitialCurrent=0  Capacitance=1e-6  Setx0=off  InitialVoltage=0  Measurements=None
  Series RLC Branch3 : spsSeriesRLCBranchLib/Series RLC Branch  LConnTagsString=__new0  RConnTagsString=__new0  BranchType=RL  Resistance=R  Inductance=L  SetiL0=off  InitialCurrent=0  Capacitance=1e-6  Setx0=off  InitialVoltage=0  Measurements=None
  Series RLC Branch6 : spsSeriesRLCBranchLib/Series RLC Branch  LConnTagsString=__new0  RConnTagsString=__new0  BranchType=RL  Resistance=R  Inductance=L  SetiL0=off  InitialCurrent=0  Capacitance=1e-6  Setx0=off  InitialVoltage=0  Measurements=None
  A : PMIOPort  Side=Left
  a : PMIOPort  Port=2  Side=Right
  B : PMIOPort  Port=3  Side=Left
  b : PMIOPort  Port=4  Side=Right
  C : PMIOPort  Port=5  Side=Left
  c : PMIOPort  Port=6  Side=Right
  connections:
  Ground5/LConn1 -- Parallel RLC Branch5/RConn1
  Ground4/LConn1 -- Parallel RLC Branch4/RConn1
  Series RLC Branch6/RConn1 -- Parallel RLC Branch5/LConn1 -- c/RConn1
  Series RLC Branch6/LConn1 -- Parallel RLC Branch4/LConn1 -- C/RConn1
  Ground3/LConn1 -- Parallel RLC Branch3/RConn1
  Ground2/LConn1 -- Parallel RLC Branch2/RConn1
  Series RLC Branch3/RConn1 -- Parallel RLC Branch3/LConn1 -- b/RConn1
  Series RLC Branch3/LConn1 -- Parallel RLC Branch2/LConn1 -- B/RConn1
  Parallel RLC Branch1/LConn1 -- a/RConn1 -- Series RLC Branch/RConn1
  Ground/LConn1 -- Parallel RLC Branch/RConn1
  Parallel RLC Branch/LConn1 -- A/RConn1 -- Series RLC Branch/LConn1
  Ground1/LConn1 -- Parallel RLC Branch1/RConn1

== system benchmark_16bus_base_scenario/GFL IDEAL VSC3/Bridge_Model ==
  Uref : Inport
  NOT1 : Logic  Operator=NOT  IconShape=distinctive  AllPortsSameDT=off  OutDataTypeStr=boolean
  Saturation : Saturate  UpperLimit=1  LowerLimit=-1
  Step : Step  Time=Output_Delay  SampleTime=0
  Terminator : Terminator
  Three-Phase Breaker2 : spsThreePhaseBreakerLib/Three-Phase Breaker  InitialState=open  SwitchA=on  SwitchB=on  SwitchC=on  SwitchTimes="[4/60  10/60]"  External=on  BreakerResistance=1e-5*Zb  SnubberResistance=1e6  SnubberCapacitance=inf  Measurements=None
  Three-Phase Breaker3 : spsThreePhaseBreakerLib/Three-Phase Breaker  InitialState=closed  SwitchA=on  SwitchB=on  SwitchC=on  SwitchTimes="[4/60  10/60]"  External=on  BreakerResistance=1e-6*Zb  SnubberResistance=1e6  SnubberCapacitance=inf  Measurements=None
  Three-Phase Source : spsThreePhaseSourceLib/Three-Phase Source  InternalConnection=Yg  VoltagePhases=off  Voltage=Vm0*Un1  PhaseAngle=Theta_Vm0  Voltage_phases=[25e3 25e3 25e3]/sqrt(3)  PhaseAngles_phases=[0 -120 +120]  Frequency=fb  NonIdealSource=off  SpecifyImpedance=off  Resistance=0  Inductance=0  ShortCircuitLevel=100e6  BaseVoltage=VSC01_Un1  XRratio=7  BusType=swing  Pref=0.3  Qref=0  Prefabc=[10e3, 10e3, 10e3]  Qrefabc=[0, 0, 0]  Qmin=-Inf  Qmax=Inf
  Universal Bridge : spsUniversalBridgeLib/Universal Bridge  Arms=3  SnubberResistance=1e5  SnubberCapacitance=inf  Device=Average-model based VSC  Ron=1e-3  Lon=0  ForwardVoltages="[  0  0  ]"  ForwardVoltage=0  GTOparameters=[ 10e-6 , 20e-6 ]  IGBTparameters=[ 1e-6 , 2e-6 ]  Measurements=None  Measurements_2=None  converterType=Rectifier
  Vdc : spsVoltageMeasurementLib/Voltage Measurement  PhasorSimulation=off  OutputType=Complex  PSBequivalent=0
  mp3 : Gain  Gain=2/Udcn
  PhA : PMIOPort  Side=Right
  PhB : PMIOPort  Port=2  Side=Right
  PhC : PMIOPort  Port=3  Side=Right
  Vdc+ : PMIOPort  Port=4  Side=Left
  Vdc- : PMIOPort  Port=5  Side=Left
  wires:
  Vdc/1 -> Terminator/1
  Uref/1 -> mp3/1
  mp3/1 -> Saturation/1
  NOT1/1 -> Three-Phase Breaker3/1
  Saturation/1 -> Universal Bridge/1
  Step/1 -> NOT1/1, Three-Phase Breaker2/1
  connections:
  Vdc-/RConn1 -- Universal Bridge/RConn2 -- Vdc/LConn2
  Vdc+/RConn1 -- Universal Bridge/RConn1 -- Vdc/LConn1
  PhC/RConn1 -- Three-Phase Breaker3/LConn3 -- Three-Phase Breaker2/LConn3
  PhB/RConn1 -- Three-Phase Breaker3/LConn2 -- Three-Phase Breaker2/LConn2
  PhA/RConn1 -- Three-Phase Breaker3/LConn1 -- Three-Phase Breaker2/LConn1
  Three-Phase Breaker2/RConn3 -- Universal Bridge/LConn3
  Three-Phase Breaker2/RConn2 -- Universal Bridge/LConn2
  Three-Phase Breaker2/RConn1 -- Universal Bridge/LConn1
  Three-Phase Breaker3/RConn1 -- Three-Phase Source/RConn1
  Three-Phase Breaker3/RConn2 -- Three-Phase Source/RConn2
  Three-Phase Breaker3/RConn3 -- Three-Phase Source/RConn3
